simulink model "motor"  (R2018a)
settings: Solver=VariableStepAuto  StartTime=0.0  StopTime=10.0  RelTol=1e-3
values from neighbouring files (symbols this model uses):
  D = 1e-3 / 8100 * 60 / (2 * pi) + d    [parameters.m]
  J = 5.6e-7 + j    [parameters.m]
  Ke = 1.4e-3 * 60 / (2 * pi)    (= 0.0133690152197)    [parameters.m]
  Km = 13.4e-3    (= 0.0134)    [parameters.m]
  L = 65e-6    (= 6.5e-05)    [parameters.m]
  lambda = 10    [parameters.m]
  R = 1.9    [parameters.m]
  r = 0.03    [parameters.m]
undefined symbols (not defined in the file or in its folder): sigbuilder_block
libraries: simulink x1
settings Model: Creator=loywong  LastModifiedBy=loywong

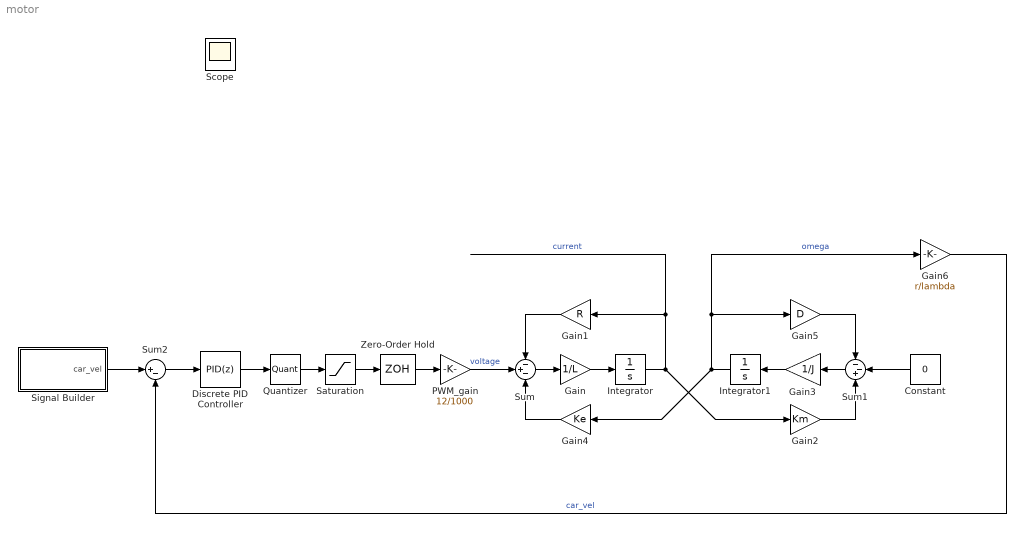
== system motor ==
  Constant : Constant  Value=0
  Discrete PID Controller : simulink/Continuous/PID Controller  Controller=PID  TimeDomain=Discrete-time  SampleTime=0.001  IntegratorMethod=Forward Euler  FilterMethod=Forward Euler  Form=Parallel  UseFilter=on  ControllerParametersSource=internal  P=711.701070017023  I=23206.1340361398  D=1.5869270531893  N=81.4683903751308  InitialConditionSource=internal  InitialConditionForIntegrator=0  InitialConditionForFilter=0  ExternalReset=none  LimitOutput=off  UpperSaturationLimit=inf  LowerSaturationLimit=-inf  LinearizeAsGain=off  AntiWindupMode=none  Kb=1  TrackingMode=off  Kt=1  PParamMin=[]  PParamMax=[]  IParamMin=[]  IParamMax=[]  DParamMin=[]  DParamMax=[]  NParamMin=[]  NParamMax=[]  KbParamMin=[]  KbParamMax=[]  KtParamMin=[]  KtParamMax=[]  POutMin=[]  POutMax=[]  IOutMin=[]  IOutMax=[]  DOutMin=[]  DOutMax=[]  NOutMin=[]  NOutMax=[]  KbOutMin=[]  KbOutMax=[]  KtOutMin=[]  KtOutMax=[]  IntegratorOutMin=[]  IntegratorOutMax=[]  FilterOutMin=[]  FilterOutMax=[]  SumOutMin=[]  SumOutMax=[]  SumI1OutMin=[]  SumI1OutMax=[]  SumI2OutMin=[]  SumI2OutMax=[]  SumI3OutMin=[]  SumI3OutMax=[]  SumDOutMin=[]  SumDOutMax=[]  SaturationOutMin=[]  SaturationOutMax=[]  IntegratorContinuousStateAttributes=''  IntegratorStateMustResolveToSignalObject=off  IntegratorRTWStateStorageClass=Auto  FilterContinuousStateAttributes=''  FilterStateMustResolveToSignalObject=off  FilterRTWStateStorageClass=Auto  DifferentiatorICPrevScaledInput=0  DifferentiatorOutMin=[]  DifferentiatorOutMax=[]  FilterDiffOutCoefMin=[]  FilterDiffOutCoefMax=[]  SumDenOutMin=[]  SumDenOutMax=[]  SumNumOutMin=[]  SumNumOutMax=[]  ReciprocalOutMin=[]  ReciprocalOutMax=[]  DivideOutMin=[]  DivideOutMax=[]  TunerSelectOption=Transfer Function Based (PID Tuner App)
  Gain : Gain  Gain=1/L
  Gain1 : Gain  Gain=R
  Gain2 : Gain  Gain=Km
  Gain3 : Gain  Gain=1/J
  Gain4 : Gain  Gain=Ke
  Gain5 : Gain  Gain=D
  Gain6 : Gain  Gain=r/lambda
  Integrator : Integrator
  Integrator1 : Integrator
  PWM_gain : Gain  Gain=12/1000
  Quantizer : Quantizer  QuantizationInterval=1
  Saturation : Saturate  UpperLimit=1000  LowerLimit=-1000
  Signal Builder : Subsystem  Tag=STV Subsys  LoadFcn=sigbuilder_block('load');  StartFcn=sigbuilder_block('start');  StopFcn=sigbuilder_block('stop');  ClipboardFcn=sigbuilder_block('clipboard');  mask(Sigbuilder block){tuvar=[0:10]}
      mask help: Simulink:masks:SigbuilderBlock_MD
      mask init:
      | if ~strcmp(get_param(bdroot(gcbh),'SimulationStatus'),'stopped') tuvar = sigbuilder_block('maskInit'); end
      settings: CopyFcn=sigbuilder_block('copy');  DeleteFcn=sigbuilder_block('delete');  ModelCloseFcn=sigbuilder_block('modelClose');  PreSaveFcn=sigbuilder_block('preSave');  PauseFcn=sigbuilder_block('pause');  ContinueFcn=sigbuilder_block('continue');  NameChangeFcn=sigbuilder_block('namechange');  OpenFcn=sigbuilder_block('open',[296 242 700 516 ]);  CloseFcn=sigbuilder_block('close');
      mask Display: plot(0, 0, 100, 100,[2, 2, 32, 32, 2], [68, 8, 8, 68, 68],[32, 2], [38, 38], [32, 19, 2],[53, 60, 44], [32, 17, 17, 2],[16, 16, 31, 31]);txt = getActiveGroup(gcbh);text(2, 100, txt,'verticalAlignment', 'top');
  Sum : Sum  Inputs=-+-
  Sum1 : Sum  Inputs=--+
  Sum2 : Sum  Inputs=|+-
  Zero-Order Hold : ZeroOrderHold  SampleTime=-1
  Scope : Scope
  wires:
  Gain5/1 -> Sum1/1
  Gain1/1 -> Sum/1
  Gain/1 -> Integrator/1
  Sum/1 -> Gain/1
  Constant/1 -> Sum1/2
  Sum1/1 -> Gain3/1
  Integrator/1 -> Gain2/1, Gain1/1  "current"
  Gain2/1 -> Sum1/3
  Gain3/1 -> Integrator1/1
  Gain4/1 -> Sum/3
  Integrator1/1 -> Gain6/1, Gain5/1, Gain4/1  "omega"
  Gain6/1 -> Sum2/2  "car_vel"
  PWM_gain/1 -> Sum/2  "voltage"
  Quantizer/1 -> Saturation/1
  Discrete PID Controller/1 -> Quantizer/1
  Zero-Order Hold/1 -> PWM_gain/1
  Saturation/1 -> Zero-Order Hold/1
  Sum2/1 -> Discrete PID Controller/1
  Signal Builder/1(car_vel) -> Sum2/1

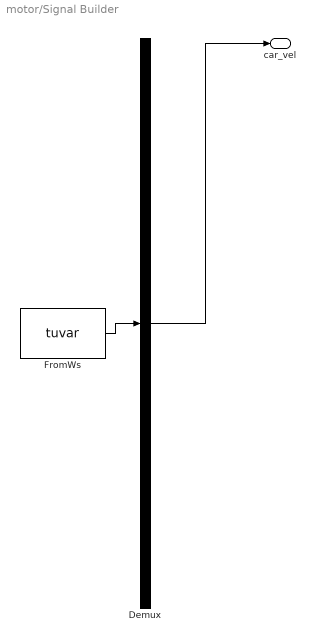
== system motor/Signal Builder ==
  Demux : Demux  Tag=STV Demux  Outputs=1
  FromWs : FromWorkspace  Tag=STV FromWs  VariableName=tuvar  SampleTime=0
      SigBuilderData=|
      | common.afterFinalStr = 'Extrapolate'
      | common.sampleTime = 0
      | dataSet.timeRange = [0 10]
      | dataSet.name = 'Group 1'
      | sbobj.Groups.Name = 'Group 1'
      | sbobj.Groups.Signals.Name = 'car_vel'
      | sbobj.Groups.Signals.XData = [0 1 1 2 2 3 3 4 4 5 6 8 9 10]
      | sbobj.Groups.Signals.YData = [0 0 1.5 1.5 0 0 -1.5 -1.5 0 0 2 -2 0 0]
  car_vel : Outport  Tag=STV Outport
  wires:
  Demux/1 -> car_vel/1
  FromWs/1 -> Demux/1
